simulink model "model"  (R2019b)
settings: Solver=VariableStepAuto  StartTime=0.0  StopTime=10.0  RelTol=1e-3
libraries: fuzblock x4
settings Model: Creator=robbie  LastModifiedBy=conor

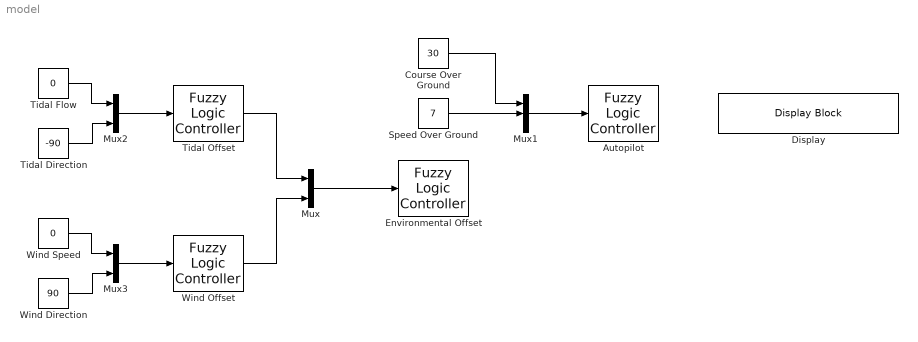
== system model ==
  Autopilot : fuzblock/Fuzzy Logic  Controller  FIS='autopilot.fis'  OutputSampleNumber=101  DataType=double  FuzzifiedInputs=off  RuleFiringStrengths=off  RuleOutputs=off  AggregatedOutputs=off  SimulateUsing=Interpreted execution  OutOfRangeInputValueMessage=warning  NoRuleFiredMessage=warning  EmptyOutputFuzzySetMessage=warning
  Course Over Ground : Constant  Value=30
  Display : DisplayBlock  LabelPosition=Hide  Format=short  Transparency=1
  Environmental Offset : fuzblock/Fuzzy Logic  Controller  FIS='environmental.fis'  OutputSampleNumber=101  DataType=double  FuzzifiedInputs=off  RuleFiringStrengths=off  RuleOutputs=off  AggregatedOutputs=off  SimulateUsing=Interpreted execution  OutOfRangeInputValueMessage=warning  NoRuleFiredMessage=warning  EmptyOutputFuzzySetMessage=warning
  Mux : Mux  Inputs=2
  Mux1 : Mux  Inputs=3
  Mux2 : Mux  Inputs=2
  Mux3 : Mux  Inputs=2
  Speed Over Ground : Constant  Value=7
  Tidal Direction : Constant  Value=-90
  Tidal Flow : Constant  Value=0
  Tidal Offset : fuzblock/Fuzzy Logic  Controller  FIS='tide.fis'  OutputSampleNumber=101  DataType=double  FuzzifiedInputs=off  RuleFiringStrengths=off  RuleOutputs=off  AggregatedOutputs=off  SimulateUsing=Interpreted execution  OutOfRangeInputValueMessage=warning  NoRuleFiredMessage=warning  EmptyOutputFuzzySetMessage=warning
  Wind Direction : Constant  Value=90
  Wind Offset : fuzblock/Fuzzy Logic  Controller  FIS='wind.fis'  OutputSampleNumber=101  DataType=double  FuzzifiedInputs=off  RuleFiringStrengths=off  RuleOutputs=off  AggregatedOutputs=off  SimulateUsing=Interpreted execution  OutOfRangeInputValueMessage=warning  NoRuleFiredMessage=warning  EmptyOutputFuzzySetMessage=warning
  Wind Speed : Constant  Value=0
  wires:
  Tidal Offset/1 -> Mux/1
  Wind Offset/1 -> Mux/2
  Mux/1 -> Environmental Offset/1
  Mux1/1 -> Autopilot/1
  Tidal Flow/1 -> Mux2/1
  Tidal Direction/1 -> Mux2/2
  Mux2/1 -> Tidal Offset/1
  Wind Direction/1 -> Mux3/2
  Wind Speed/1 -> Mux3/1
  Mux3/1 -> Wind Offset/1
  Speed Over Ground/1 -> Mux1/2
  Course Over Ground/1 -> Mux1/1
